simulink model "DCMotor"  (R2013a)
settings: Solver=VariableStepDiscrete  StartTime=0.0  StopTime=3600  FixedStep=0.002  RelTol=1e-3
settings Model: ExtModeTrigDuration=5000  Creator=Admin  LastModifiedBy=Admin
settings SolverCC: PositivePriorityOrder=on
settings DebuggingCC: SolverPrmCheckMsg=none
settings RTWCC: SystemTargetFile=quarc_win64.tlc  TemplateMakefile=quarc_default_tmf  Description=QUARC Win64 Target  ProcessScript=quarc_win64_make_rtw_hook
settings STFCustomTargetCC: TargetPreCompLibLocation=C:\PROGRA~3\QUARC\lib\2013a\win64\release  GeneratePreprocessorConditionals=Disable all  CombineOutputUpdateFcns=on  SystemTargetFile=quarc_win64.tlc
settings GRTTargetCC: TargetPreCompLibLocation=C:\PROGRA~3\QUARC\lib\2013a\win64\release  ParMdlRefBuildCompliant=off  CompOptLevelCompliant=off  ConcurrentExecutionCompliant=off  MatFileLogging=off  ExtMode=on  ExtModeMexFile=quarc_comm

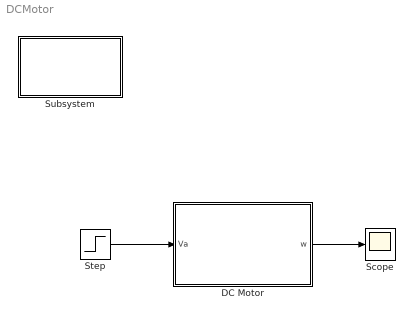
== system DCMotor ==
  DC Motor : Subsystem  mask{Ts=0.05}
      mask prompts: Ts "Sample time"
      mask Display:
      | image('img/dcmotor.png')
      | port_label('output', 1, 'w')
      | port_label('input', 1, 'Va')
  Scope : Scope
      settings: YMin=0  YMax=4
  Step : Step  After=6  SampleTime=0.05
  Subsystem : Subsystem
      mask Display: image('img/logo.png')
  wires:
  Step/1 -> DC Motor/1(Va)
  DC Motor/1(w) -> Scope/1

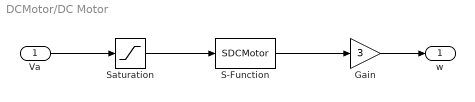
== system DCMotor/DC Motor ==
  Va : Inport
  Gain : Gain  Gain=3  SampleTime=Ts
  S-Function : S-Function  FunctionName=SDCMotor  Parameters=Ts  EnableBusSupport=off
  Saturation : Saturate  UpperLimit=10  LowerLimit=0  SampleTime=Ts
  w : Outport
  wires:
  S-Function/1 -> Gain/1
  Va/1 -> Saturation/1
  Saturation/1 -> S-Function/1
  Gain/1 -> w/1

== system DCMotor/Subsystem ==
